simulink model "ex1_2015"  (Simulink 8.6)
settings: Solver=VariableStepAuto  SolverMode=SingleTasking  StartTime=0.0  StopTime=10.0  RelTol=1e-3
values from neighbouring files (symbols this model uses):
  a = 1    [ex1_ss.m]    (also in ex2_ss.m = [0 1 0 0; ex3_ss.m = [2 3; 1 4])
  b = 1    [ex1_ss.m]    (also in ex2_ss.m = [0;1;0;-2]; ex3_ss.m = [1 0;0 1])
  c = 1    [ex1_ss.m]    (also in ex2_ss.m = [1 0 0 0]; ex3_ss.m = [1 0;0 1])
  d = 0    [ex1_ss.m]    (also in ex2_ss.m; ex3_ss.m)
  K = place(Aa,Ba,polos)    [ex1_ss.m]    (also in ex2_ss.m; ex3_ss.m)
settings Model: Creator=Sergio  LastModifiedBy=Sergio
settings DataIOCC: LimitDataPoints=off  SaveFormat=Dataset  SignalLoggingSaveFormat=Dataset  ReturnWorkspaceOutputs=on
settings OptimizationCC: ExpressionDepthLimit=128
settings DebuggingCC: UnderspecifiedInitializationDetection=Simplified  MergeDetectMultiDrivingBlocksExec=error  SolverPrmCheckMsg=none  FcnCallInpInsideContextMsg=EnableAllAsError  AllowSymbolicDim=on  StateNameClashWarn=none  SFUnexpectedBacktrackingDiag=error  SFNoUnconditionalDefaultTransitionDiag=error
settings HardwareCC: ProdBitPerPointer=64  ProdLargestAtomicFloat=Float  ProdIntDivRoundTo=Zero  ProdEndianess=LittleEndian  ProdWordSize=64  ProdHWDeviceType=Intel->x86-64 (Windows64)
settings ModelReferenceCC: PropagateSignalLabelsOutOfModel=on
settings SFSimCC: SimUseLocalCustomCode=on
settings RTWCC: RTWUseLocalCustomCode=on
settings GRTTargetCC: TargetLangStandard=C99 (ISO)  CombineOutputUpdateFcns=on  GRTInterface=off
settings ConfigComp: CovMetricSettings=dwe  CovHtmlReporting=off  CovSaveCumulativeToWorkspaceVar=off  CovSaveSingleToWorkspaceVar=off  CovExternalEMLEnable=on

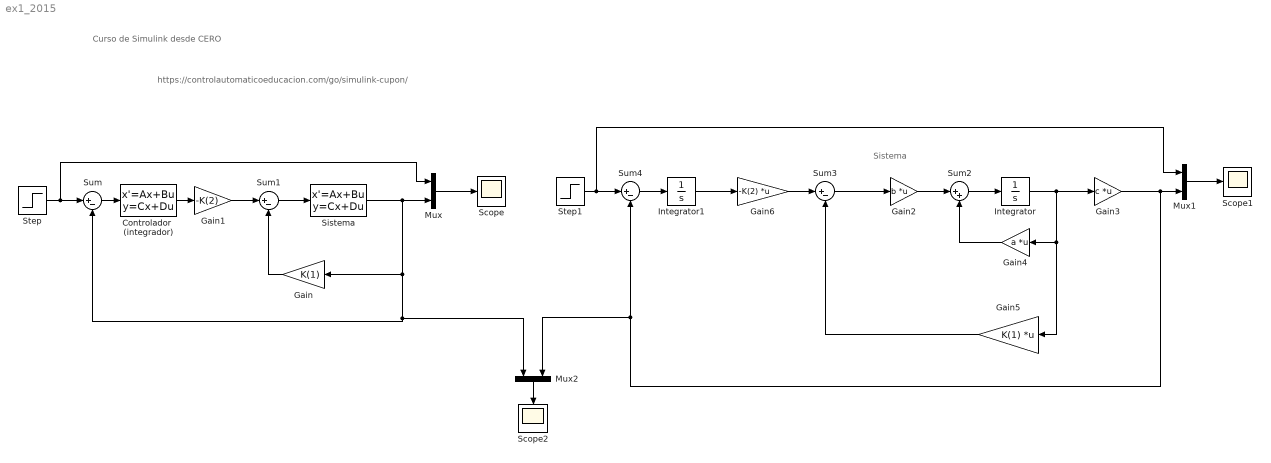
== system ex1_2015 ==
  note: https://controlautomaticoeducacion.com/go/simulink-cupon/
  note: Curso de Simulink desde CERO
  note: Sistema
  Controlador  (integrador) : StateSpace  A=0  D=0  X0=0
  Gain : Gain  Gain=K(1)
  Gain1 : Gain  Gain=-K(2)
  Gain2 : Gain  Gain=b  Multiplication=Matrix(K*u)
  Gain3 : Gain  Gain=c  Multiplication=Matrix(K*u)
  Gain4 : Gain  Gain=a  Multiplication=Matrix(K*u)
  Gain5 : Gain  Gain=K(1)  Multiplication=Matrix(K*u)
  Gain6 : Gain  Gain=-K(2)  Multiplication=Matrix(K*u)
  Integrator : Integrator
  Integrator1 : Integrator
  Mux : Mux  Inputs=2
  Mux1 : Mux  Inputs=2
  Mux2 : Mux  Inputs=2
  Scope : Scope
  Scope1 : Scope
  Scope2 : Scope
  Sistema : StateSpace  A=a  B=b  C=c  D=d  X0=0
  Step : Step  SampleTime=0
  Step1 : Step  SampleTime=0
  Sum{,1,3..4} (4 alike) : Sum  Inputs=|+-
  Sum2 : Sum  Inputs=|++
  wires:
  Gain/1 -> Sum1/2
  Sum1/1 -> Sistema/1
  Controlador  (integrador)/1 -> Gain1/1
  Step/1 -> Mux/1, Sum/1
  Sum/1 -> Controlador  (integrador)/1
  Mux/1 -> Scope/1
  Gain1/1 -> Sum1/1
  Sistema/1 -> Mux/2, Gain/1, Mux2/1, Sum/2
  Integrator/1 -> Gain3/1, Gain5/1, Gain4/1
  Gain4/1 -> Sum2/2
  Sum2/1 -> Integrator/1
  Gain2/1 -> Sum2/1
  Sum3/1 -> Gain2/1
  Step1/1 -> Mux1/1, Sum4/1
  Sum4/1 -> Integrator1/1
  Integrator1/1 -> Gain6/1
  Gain6/1 -> Sum3/1
  Gain5/1 -> Sum3/2
  Gain3/1 -> Mux2/2, Sum4/2, Mux1/2
  Mux1/1 -> Scope1/1
  Mux2/1 -> Scope2/1
